simulink model "Mostar"  (Simulink 9.2)
settings: Solver=ode23s  StartTime=0  StopTime=70  FixedStep=0.01  RelTol=0.001  EnableMultiTasking=on
libraries: fmu_me_lib x1
settings Model: Creator=Tin Rabuzin  LastModifiedBy=meagh
settings DataIOCC: SignalLoggingSaveFormat=Dataset  OutputSaveName=simout  OutputOption=SpecifiedOutputTimes  OutputTimes=[0:0.05:70]
settings OptimizationCC: ExpressionDepthLimit=2147483647
settings DebuggingCC: FcnCallInpInsideContextMsg=error
settings GRTTargetCC: CombineOutputUpdateFcns=on  GRTInterface=off

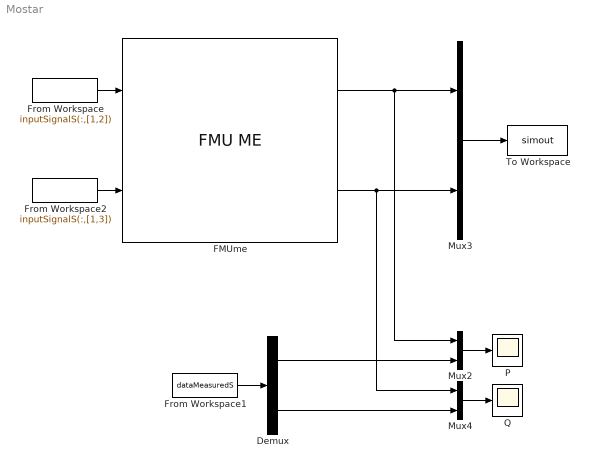
== system Mostar ==
  Demux : Demux  Outputs=2
  FMUme : fmu_me_lib/FMU ME  Description=Simulates an FMU for Model Exchange 1.0 or Model Exchange 2.0.  dummy=0
  From Workspace : FromWorkspace  VariableName=inputSignalS(:,[1,2])  SampleTime=0  OutputAfterFinalValue=Holding final value
  From Workspace1 : FromWorkspace  VariableName=dataMeasuredS  SampleTime=0
  From Workspace2 : FromWorkspace  VariableName=inputSignalS(:,[1,3])  SampleTime=0  OutputAfterFinalValue=Holding final value
  Mux2 : Mux  Inputs=2
  Mux3 : Mux  Inputs=2
  Mux4 : Mux  Inputs=2
  P : Scope
  Q : Scope
  To Workspace : ToWorkspace  VariableName=simout  SaveFormat=Structure With Time  SampleTime=-1
  wires:
  From Workspace1/1 -> Demux/1
  Demux/1 -> Mux2/2
  Mux3/1 -> To Workspace/1
  Mux2/1 -> P/1
  Mux4/1 -> Q/1
  FMUme/1 -> Mux2/1, Mux3/1
  From Workspace/1 -> FMUme/1
  From Workspace2/1 -> FMUme/2
  Demux/2 -> Mux4/2
  FMUme/2 -> Mux4/1, Mux3/2
